simulink model "GitAffineFormationDelayInput"  (R2020b)
settings: Solver=ode4  StartTime=0.0  StopTime=50  FixedStep=0.01  RelTol=1e-3
(part 2 of 2)

== matlab function GitAffineFormationDelayInput/Subsystem12/MATLAB Function ==
  data: T input; outputArg1 output; outputArg2 output; vxx input; A input; W input; C input
function [outputArg1,outputArg2] = fcn_leaderV1(T,vxx,A,W,C)
current_time = T;
a=A;
w=W;
c=C;
vx=vxx;
vy = a*cos(w*current_time)+c;
outputArg1 = vx;
outputArg2 = vy;
end

== matlab function GitAffineFormationDelayInput/Subsystem13/MATLAB Function1 ==
  data: T input; outputArg1 output; outputArg2 output; vxx input; A input; W input; C input
function [outputArg1,outputArg2] = fcn_leaderV2(T,vxx,A,W,C)
current_time = T;
a=A;
w=W;
c=C;
vx=vxx;
vy = a*cos(w*current_time)+c;
outputArg1 = vx;
outputArg2 = vy;
end

== matlab function GitAffineFormationDelayInput/Subsystem14/MATLAB Function2 ==
  data: T input; outputArg1 output; outputArg2 output; vxx input; A input; W input; C input
function [outputArg1,outputArg2] = fcn_leaderV3(T,vxx,A,W,C)
current_time = T;
a=A;
w=W;
c=C;
vx=vxx;
vy = a*cos(w*current_time)+c;
outputArg1 = vx;
outputArg2 = vy;
end

== matlab function GitAffineFormationDelayInput/Subsystem/MATLAB Function3 ==
  data: v input; vx output size=1; p input; vy output size=1; kaa input; kbb input
function [vx,vy] = fcn_followerV4(v,p,kaa,kbb)

reV=zeros(2,9);
reP=zeros(2,9);
reV=reshape(v,2,9);
reP=reshape(p,2,9);


ka=kaa;
kb=kbb;
vx4=0;
vy4=0;

%% 9cars
nodenum=9;
leaderNum=3;
neighborMat=zeros(nodenum,nodenum);
neighborMat(1,2)=1;neighborMat(1,3)=1;neighborMat(1,8)=1;neighborMat(1,9)=1;
neighborMat(2,4)=1;neighborMat(2,7)=1;
neighborMat(3,5)=1;neighborMat(3,6)=1;neighborMat(3,4)=1;neighborMat(2,5)=1;
neighborMat(4,5)=1;neighborMat(4,6)=1;neighborMat(2,7)=1;neighborMat(4,7)=0;
neighborMat(5,7)=1;neighborMat(5,8)=0;neighborMat(5,6)=0;
neighborMat(6,7)=1;neighborMat(6,8)=1;
neighborMat(7,9)=1;
neighborMat(8,9)=1;
m=sum(sum(neighborMat)); % number of edges
neighborMat=neighborMat+neighborMat';
stressMat=[-0.438878870659884,0.292585913773256,0.292585913773256,0,0,0,0,-0.0731464784433140,-0.0731464784433141;0.292585913773256,-0.615360326958201,0,0.420303051109364,-0.0673401385127307,0,-0.0301884994116881,0,0;0.292585913773256,0,-0.615360326958201,-0.0673401385127306,0.420303051109363,-0.0301884994116881,0,0,0;0,0.420303051109364,-0.0673401385127306,-0.703215455187769,-0.00271037000549659,0.352962912596633,0,0,0;0,-0.0673401385127307,0.420303051109363,-0.00271037000549659,-0.703215455187768,0,0.352962912596632,0,0;0,0,-0.0301884994116881,0.352962912596633,0,-0.607698639186239,-0.00766168777196264,0.292585913773257,0;0,-0.0301884994116881,0,0,0.352962912596632,-0.00766168777196264,-0.607698639186238,0,0.292585913773256;-0.0731464784433140,0,0,0,0,0.292585913773257,0,-0.402305631438228,0.182866196108285;-0.0731464784433141,0,0,0,0,0,0.292585913773256,0.182866196108285,-0.402305631438227];

%%
for j=1:nodenum 
    if neighborMat(4,j)==1 && j~=4
        omegaij=stressMat(4,j);
        vx4=vx4-ka*kb*omegaij*(reP(1,4)-reP(1,j))-kb*omegaij*(reV(1,4)-reV(1,j));
        vy4=vy4-ka*kb*omegaij*(reP(2,4)-reP(2,j))-kb*omegaij*(reV(2,4)-reV(2,j));
    end
end
vx4=vx4+reV(1,4);
vy4=vy4+reV(2,4);


vx = vx4;
vy = vy4;
